simulink model "PIDControllerTest"  (R2025b)
settings: Solver=FixedStepAuto  StartTime=0.0  StopTime=inf  FixedStep=.01  RelTol=1e-3
settings Model: Creator=talles  LastModifiedBy=ajax

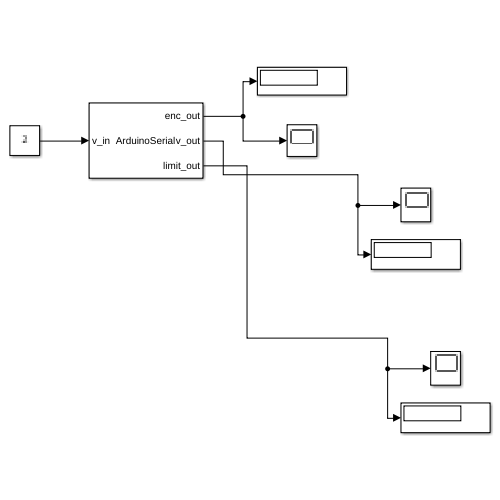
[thumbnail: Simulink's stored preview of the top-level diagram]
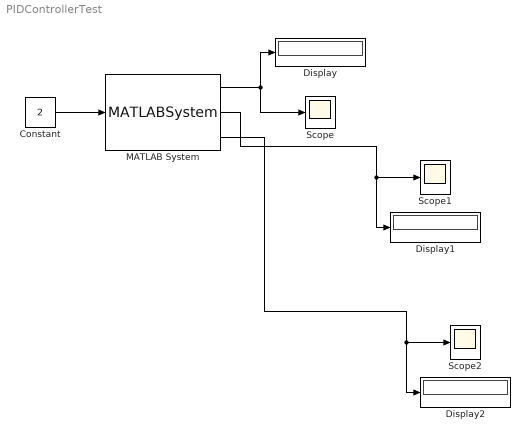
== system PIDControllerTest ==
  Constant : Constant  Value=2
  Display : Display
  Display1 : Display
  Display2 : Display
  MATLAB System : MATLABSystem  System=ArduinoSerial  COMPort=/dev/ttyACM0  BaudRate=115200  TargetPos=500  Direction=Positive  SimulateUsing=Code generation
      mask Type: ArduinoSerial
  Scope : Scope
      settings: ActiveDisplayYMinimum=1  ActiveDisplayYMaximum=3
  Scope1 : Scope
      settings: ActiveDisplayYMinimum=-6.0034594760493682  ActiveDisplayYMaximum=14.706273819701902
  Scope2 : Scope
      settings: ActiveDisplayYMinimum=-6.0034594760493682  ActiveDisplayYMaximum=14.706273819701902  DataLoggingVariableName=ScopeData2
  wires:
  MATLAB System/1 -> Scope/1, Display/1
  MATLAB System/2 -> Display1/1, Scope1/1
  Constant/1 -> MATLAB System/1
  MATLAB System/3 -> Display2/1, Scope2/1
